simulink model "SimParking"  (R2017b)
settings: Solver=VariableStepAuto  StartTime=0.0  StopTime=1761  RelTol=1e-3
libraries: neural x1111
(part 2 of 60)

== system SimParking/10D- 100 100 100N/Layer 2 ==
  "a{1} " : Inport  PortDimensions=100  SampleTime=1
      mask Display: e = 0.06;c1 = [120 230 180]/255;c2 = ([120 230 180]+0)/(256+128);c3 = ([120 230 180]+128)/(256+128);patch([0 1 1 0],[0 0 1 1],c1);patch([0 1 1 1-e 1-e 0+e],[0 0 1 1-e 0+e 0+e],c2);patch([0 0 1 1-e 0+e 0+e],[0 1 1 1-e 1-e 0+e],c3);plot([0 1 1 0 0],[0 0 1 1 0]);
  Delays 1 : Subsystem
      mask Display: e = 0.06;c1 = [120 150 230]/255;c2 = ([120 150 230]+0)/383;c3 = ([120 150 230]+128)/383;patch([0 1 1 0],[0 0 1 1],c1);patch([0 1 1 1-e 1-e 0+e],[0 0 1 1-e 0+e 0+e],c2);patch([0 0 1 1-e 0+e 0+e],[0 1 1 1-e 1-e 0+e],c3);plot([0 1 1 0 0],[0 0 1 1 0]);disp('0');
  "LW{2,1}" : Subsystem
      mask Display: e = 0.06;c1 = [120 150 230]/255;c2 = ([120 150 230]+0)/383;c3 = ([120 150 230]+128)/383;patch([0 1 1 0],[0 0 1 1],c1);patch([0 1 1 1-e 1-e 0+e],[0 0 1 1-e 0+e 0+e],c2);patch([0 0 1 1-e 0+e 0+e],[0 1 1 1-e 1-e 0+e],c3);plot([0 1 1 0 0],[0 0 1 1 0]);disp('W');
  "b{2}" : Constant  Value=[1.506519516441978456811057185404933989048004150390625;-1.4371919272699462677422843626118265092372894287109375;1.4557843120845770368276816952857188880443572998046875;1.398256717805032689483368812943808734416961669921875;-1.355726258601539502279820226249285042285919189453125;1.359587166719958162275361246429383754730224609375;-1.3155039337803986487784868586459197103977203369140625;-1.3165404698274996153628535466850735247135162353515625;-1.308071637947867404960788917378522455692291259765625;1.27497404400224123577345380908809602260589599609375;1.21468909644321598761962377466261386871337890625;1.1384788543866457555253646205528639256954193115234375;1.0939944737098141747111412769299931824207305908203125;1.1256588211524605203095461547491140663623809814453125;-1.0383506087646006132985121439560316503047943115234375;-1.0161104044606033003361744704307056963443756103515625;-1.0127147984754660825501559884287416934967041015625;0.981450719068787780230422868044115602970123291015625;0.96418217538418382606124623634968884289264678955078125;-0.93556041399205736031063906921190209686756134033203125;-0.87753459394353339195760099755716510117053985595703125;0.87923441768039711785576173497247509658336639404296875;-0.8381966651892593933581565579515881836414337158203125;-0.7681328722554023880064733020844869315624237060546875;-0.75124322279230348886613910508458502590656280517578125;-0.77210854445230181486437004423351027071475982666015625;-0.71873920784606692979679110067081637680530548095703125;-0.70857184198599154623110507600358687341213226318359375;0.6807460268837750572146205740864388644695281982421875;-0.66075686590633697647945155040360987186431884765625;0.62103296432244536884326180370408110320568084716796875;-0.56357924925441860164454510595533065497875213623046875;0.5427900564652194947967700500157661736011505126953125;0.5194764137396343794961239836993627250194549560546875;-0.433960890913997643369981460637063719332218170166015625;0.4821967486735594388136405541445128619670867919921875;0.374432721983393002052054043815587647259235382080078125;-0.37755478669698827598466550625744275748729705810546875;-0.286324330953135197663783628740929998457431793212890625;-0.325139756308971794585005454791826196014881134033203125;0.33221529164236185405201240428141318261623382568359375;-0.1969409792129176162145398620850755833089351654052734375;-0.313389016592093339053093359325430355966091156005859375;-0.192144639089638025186701497659669257700443267822265625;0.2085748723544801064289089254089049063622951507568359375;0.132020705406266258830072501950780861079692840576171875;0.061838232194021347520873632674920372664928436279296875;0.047869259779082858063947725213438388891518115997314453125;-0.006209755679524676941216654313393519259989261627197265625;0.0092266532370322180967026071130021591670811176300048828125;0.004075476244258154252808612483249817159958183765411376953125;-0.06655675450056099118345542819952243007719516754150390625;0.099658129876597112417613288926077075302600860595703125;0.1334403996895525690291606224491260945796966552734375;0.10912476773787938011395226567401550710201263427734375;0.193006691977488042955002356393379159271717071533203125;-0.1454527881073393869026944003053358756005764007568359375;0.185461909127874247094069914965075440704822540283203125;0.2951347935264607702521288956631906330585479736328125;0.3158668243089579608096073570777662098407745361328125;0.294566160388877007481056580218137241899967193603515625;0.380210240619695938324440476208110339939594268798828125;-0.410584596708548243970682278813910670578479766845703125;0.36024445553864425928480841321288608014583587646484375;0.44824097005917129532548415227211080491542816162109375;0.469655642441448251123148338592727668583393096923828125;0.4462810592999779668588189451838843524456024169921875;-0.50698818603659467907363023186917416751384735107421875;0.53901197267530120971201768043101765215396881103515625;-0.54413527250999960127586518865427933633327484130859375 ...(+1616 chars)]
      mask Display: e = 0.06;c1 = [120 150 230]/255;c2 = ([120 150 230]+0)/383;c3 = ([120 150 230]+128)/383;patch([0 1 1 0],[0 0 1 1],c1);patch([0 1 1 1-e 1-e 0+e],[0 0 1 1-e 0+e 0+e],c2);patch([0 0 1 1-e 0+e 0+e],[0 1 1 1-e 1-e 0+e],c3);plot([0 1 1 0 0],[0 0 1 1 0]);disp('b');
  netsum : Sum  Inputs=2  SaturateOnIntegerOverflow=on  InputSameDT=on  OutDataTypeStr=Inherit: Same as first input
      mask Display: e = 0.06;c1 = [120 150 230]/255;c2 = ([120 150 230]+0)/383;c3 = ([120 150 230]+128)/383;patch([0 1 1 0],[0 0 1 1],c1);patch([0 1 1 1-e 1-e 0+e],[0 0 1 1-e 0+e 0+e],c2);patch([0 0 1 1-e 0+e 0+e],[0 1 1 1-e 1-e 0+e],c3);plot([0 1 1 0 0],[0 0 1 1 0]);disp('+');
  tansig : neural/Transfer Functions/tansig
  "a{2}" : Outport  InitialOutput=[0;0;0;0;0;0;0;0;0;0;0;0;0;0;0;0;0;0;0;0;0;0;0;0;0;0;0;0;0;0;0;0;0;0;0;0;0;0;0;0;0;0;0;0;0;0;0;0;0;0;0;0;0;0;0;0;0;0;0;0;0;0;0;0;0;0;0;0;0;0;0;0;0;0;0;0;0;0;0;0;0;0;0;0;0;0;0;0;0;0;0;0;0;0;0;0;0;0;0;0]
      mask Display: e = 0.06;c1 = [120 230 180]/255;c2 = ([120 230 180]+0)/(256+128);c3 = ([120 230 180]+128)/(256+128);patch([0 1 1 0],[0 0 1 1],c1);patch([0 1 1 1-e 1-e 0+e],[0 0 1 1-e 0+e 0+e],c2);patch([0 0 1 1-e 0+e 0+e],[0 1 1 1-e 1-e 0+e],c3);plot([0 1 1 0 0],[0 0 1 1 0]);
  wires:
  "a{1} "/1 -> Delays 1/1("p{2}")
  Delays 1/1("pd{2,1}") -> "LW{2,1}"/1("ad{2,1}")
  "LW{2,1}"/1("lz{2,1}") -> netsum/1
  "b{2}"/1 -> netsum/2
  netsum/1 -> tansig/1
  tansig/1 -> "a{2}"/1

== system SimParking/10D- 100 100 100N/Layer 3 ==
  "a{2} " : Inport  PortDimensions=100  SampleTime=1
      mask Display: e = 0.06;c1 = [120 230 180]/255;c2 = ([120 230 180]+0)/(256+128);c3 = ([120 230 180]+128)/(256+128);patch([0 1 1 0],[0 0 1 1],c1);patch([0 1 1 1-e 1-e 0+e],[0 0 1 1-e 0+e 0+e],c2);patch([0 0 1 1-e 0+e 0+e],[0 1 1 1-e 1-e 0+e],c3);plot([0 1 1 0 0],[0 0 1 1 0]);
  Delays 1 : Subsystem
      mask Display: e = 0.06;c1 = [120 150 230]/255;c2 = ([120 150 230]+0)/383;c3 = ([120 150 230]+128)/383;patch([0 1 1 0],[0 0 1 1],c1);patch([0 1 1 1-e 1-e 0+e],[0 0 1 1-e 0+e 0+e],c2);patch([0 0 1 1-e 0+e 0+e],[0 1 1 1-e 1-e 0+e],c3);plot([0 1 1 0 0],[0 0 1 1 0]);disp('0');
  "LW{3,2}" : Subsystem
      mask Display: e = 0.06;c1 = [120 150 230]/255;c2 = ([120 150 230]+0)/383;c3 = ([120 150 230]+128)/383;patch([0 1 1 0],[0 0 1 1],c1);patch([0 1 1 1-e 1-e 0+e],[0 0 1 1-e 0+e 0+e],c2);patch([0 0 1 1-e 0+e 0+e],[0 1 1 1-e 1-e 0+e],c3);plot([0 1 1 0 0],[0 0 1 1 0]);disp('W');
  "b{3}" : Constant  Value=[-1.4923648462887009191746301439707167446613311767578125;1.4556606612840330416958067871746607124805450439453125;-1.387278892945349451082392988610081374645233154296875;1.4028556882846070497095070095383562147617340087890625;1.345199381926466930536889776703901588916778564453125;1.3532535376566328100267355694086290895938873291015625;-1.30643871860076732360766982310451567173004150390625;-1.2638080303968048934137868855032138526439666748046875;-1.23255646908093563496322531136684119701385498046875;1.230158278997876220017815285245887935161590576171875;1.1333695566611690086489261375390924513339996337890625;-1.1083346531027700176963435296784155070781707763671875;1.11500334128624611906843711039982736110687255859375;1.0878630145011747298866566779906861484050750732421875;1.03732677279241425338796034338884055614471435546875;0.9868555056448837792260064816218800842761993408203125;-1.0240515281041224771030329065979458391666412353515625;-0.9922683117643220640502477181144058704376220703125;-0.94501809355730792550076557745342142879962921142578125;0.870249200573390613300261975382454693317413330078125;-0.8844413015848413550656914594583213329315185546875;-0.8575733682742943120302925308351404964923858642578125;0.84952879702115069449064321815967559814453125;-0.80657709043296066386830034389276988804340362548828125;0.76156012510090598244261173022096045315265655517578125;-0.7558812748899208511232927776291035115718841552734375;0.6629457722732536861798280369839631021022796630859375;-0.67179056724727337357450096533284522593021392822265625;0.64316286659681465298632474514306522905826568603515625;-0.6456362689201016191731241633533500134944915771484375;0.59942726953591651817276897418196313083171844482421875;0.531031473132824505256621705484576523303985595703125;-0.56240602810975437453322456349269486963748931884765625;-0.467483062718826669623695124755613505840301513671875;-0.4667361706627328743479665718041360378265380859375;-0.402814167048342219867862468163366429507732391357421875;0.41212203864621399507228716174722649157047271728515625;0.35396080444632815886762955415179021656513214111328125;0.3871687344655525553349662004620768129825592041015625;-0.31679874280190156721204175482853315770626068115234375;0.2611818277655080233756734742200933396816253662109375;0.238926892331456641738185453505138866603374481201171875;-0.205035418786340295493886287658824585378170013427734375;-0.2129412471957893571161690715598524548113346099853515625;-0.1596725436243604245856175793960574083030223846435546875;-0.139376121918832474033678181513096205890178680419921875;-0.11595637311078853259882492920951335690915584564208984375;0.07992718662413784980191877593824756331741809844970703125;-0.010895986891703089705085716332177980802953243255615234375;0.0183462905284579001763400896152234054170548915863037109375;2.585053176850398811890095751575557869728072546422481536865234375e-05;0.02503199263089939119453219973365776240825653076171875;-0.09852058470632696351998447426012717187404632568359375;-0.10786625805302378633410143038418027572333812713623046875;0.1860671251697297579053014260352938435971736907958984375;0.185573368129740290388696166701265610754489898681640625;-0.241184922099264398287488120331545360386371612548828125;0.20682957005122137861263809099909849464893341064453125;0.263761825941337069156844563622144050896167755126953125;-0.31559160823815213259280199054046534001827239990234375;0.33457105107667317600572687297244556248188018798828125;0.38299603176620011790731723522185347974300384521484375;-0.38103619333580873718148041007225401699542999267578125;0.414633099020468076645329347229562699794769287109375;-0.444740696637884791453387833826127462089061737060546875;-0.449524314866814489466406712381285615265369415283203125;0.474190020993898564416468843774055130779743194580078125;-0.52066741892512291567385318558081053197383880615234375;0.55714918266694135606797999571426771581172943115234375;-0.5895289389142746028227293209056369960308074951171875;-0.61193450214706912593243259834707714617252349853515625 ...(+1575 chars)]
      mask Display: e = 0.06;c1 = [120 150 230]/255;c2 = ([120 150 230]+0)/383;c3 = ([120 150 230]+128)/383;patch([0 1 1 0],[0 0 1 1],c1);patch([0 1 1 1-e 1-e 0+e],[0 0 1 1-e 0+e 0+e],c2);patch([0 0 1 1-e 0+e 0+e],[0 1 1 1-e 1-e 0+e],c3);plot([0 1 1 0 0],[0 0 1 1 0]);disp('b');
  netsum : Sum  Inputs=2  SaturateOnIntegerOverflow=on  InputSameDT=on  OutDataTypeStr=Inherit: Same as first input
      mask Display: e = 0.06;c1 = [120 150 230]/255;c2 = ([120 150 230]+0)/383;c3 = ([120 150 230]+128)/383;patch([0 1 1 0],[0 0 1 1],c1);patch([0 1 1 1-e 1-e 0+e],[0 0 1 1-e 0+e 0+e],c2);patch([0 0 1 1-e 0+e 0+e],[0 1 1 1-e 1-e 0+e],c3);plot([0 1 1 0 0],[0 0 1 1 0]);disp('+');
  tansig : neural/Transfer Functions/tansig
  "a{3}" : Outport  InitialOutput=[0;0;0;0;0;0;0;0;0;0;0;0;0;0;0;0;0;0;0;0;0;0;0;0;0;0;0;0;0;0;0;0;0;0;0;0;0;0;0;0;0;0;0;0;0;0;0;0;0;0;0;0;0;0;0;0;0;0;0;0;0;0;0;0;0;0;0;0;0;0;0;0;0;0;0;0;0;0;0;0;0;0;0;0;0;0;0;0;0;0;0;0;0;0;0;0;0;0;0;0]
      mask Display: e = 0.06;c1 = [120 230 180]/255;c2 = ([120 230 180]+0)/(256+128);c3 = ([120 230 180]+128)/(256+128);patch([0 1 1 0],[0 0 1 1],c1);patch([0 1 1 1-e 1-e 0+e],[0 0 1 1-e 0+e 0+e],c2);patch([0 0 1 1-e 0+e 0+e],[0 1 1 1-e 1-e 0+e],c3);plot([0 1 1 0 0],[0 0 1 1 0]);
  wires:
  "a{2} "/1 -> Delays 1/1("p{3}")
  Delays 1/1("pd{3,2}") -> "LW{3,2}"/1("ad{3,2}")
  "LW{3,2}"/1("lz{3,2}") -> netsum/1
  "b{3}"/1 -> netsum/2
  netsum/1 -> tansig/1
  tansig/1 -> "a{3}"/1

== system SimParking/10D- 100 100 100N/Layer 4 ==
  "a{3} " : Inport  PortDimensions=100  SampleTime=1
      mask Display: e = 0.06;c1 = [120 230 180]/255;c2 = ([120 230 180]+0)/(256+128);c3 = ([120 230 180]+128)/(256+128);patch([0 1 1 0],[0 0 1 1],c1);patch([0 1 1 1-e 1-e 0+e],[0 0 1 1-e 0+e 0+e],c2);patch([0 0 1 1-e 0+e 0+e],[0 1 1 1-e 1-e 0+e],c3);plot([0 1 1 0 0],[0 0 1 1 0]);
  Delays 1 : Subsystem
      mask Display: e = 0.06;c1 = [120 150 230]/255;c2 = ([120 150 230]+0)/383;c3 = ([120 150 230]+128)/383;patch([0 1 1 0],[0 0 1 1],c1);patch([0 1 1 1-e 1-e 0+e],[0 0 1 1-e 0+e 0+e],c2);patch([0 0 1 1-e 0+e 0+e],[0 1 1 1-e 1-e 0+e],c3);plot([0 1 1 0 0],[0 0 1 1 0]);disp('0');
  "LW{4,3}" : Subsystem
      mask Display: e = 0.06;c1 = [120 150 230]/255;c2 = ([120 150 230]+0)/383;c3 = ([120 150 230]+128)/383;patch([0 1 1 0],[0 0 1 1],c1);patch([0 1 1 1-e 1-e 0+e],[0 0 1 1-e 0+e 0+e],c2);patch([0 0 1 1-e 0+e 0+e],[0 1 1 1-e 1-e 0+e],c3);plot([0 1 1 0 0],[0 0 1 1 0]);disp('W');
  "b{4}" : Constant  Value=[0.90458221227192170399433734928607009351253509521484375;-0.09842194346834050311390029719404992647469043731689453125;-0.8300561660103167316293593103182502090930938720703125]
      mask Display: e = 0.06;c1 = [120 150 230]/255;c2 = ([120 150 230]+0)/383;c3 = ([120 150 230]+128)/383;patch([0 1 1 0],[0 0 1 1],c1);patch([0 1 1 1-e 1-e 0+e],[0 0 1 1-e 0+e 0+e],c2);patch([0 0 1 1-e 0+e 0+e],[0 1 1 1-e 1-e 0+e],c3);plot([0 1 1 0 0],[0 0 1 1 0]);disp('b');
  netsum : Sum  Inputs=2  SaturateOnIntegerOverflow=on  InputSameDT=on  OutDataTypeStr=Inherit: Same as first input
      mask Display: e = 0.06;c1 = [120 150 230]/255;c2 = ([120 150 230]+0)/383;c3 = ([120 150 230]+128)/383;patch([0 1 1 0],[0 0 1 1],c1);patch([0 1 1 1-e 1-e 0+e],[0 0 1 1-e 0+e 0+e],c2);patch([0 0 1 1-e 0+e 0+e],[0 1 1 1-e 1-e 0+e],c3);plot([0 1 1 0 0],[0 0 1 1 0]);disp('+');
  purelin : neural/Transfer Functions/purelin
  "a{4}" : Outport  InitialOutput=[0;0;0]
      mask Display: e = 0.06;c1 = [120 230 180]/255;c2 = ([120 230 180]+0)/(256+128);c3 = ([120 230 180]+128)/(256+128);patch([0 1 1 0],[0 0 1 1],c1);patch([0 1 1 1-e 1-e 0+e],[0 0 1 1-e 0+e 0+e],c2);patch([0 0 1 1-e 0+e 0+e],[0 1 1 1-e 1-e 0+e],c3);plot([0 1 1 0 0],[0 0 1 1 0]);
  wires:
  "a{3} "/1 -> Delays 1/1("p{4}")
  Delays 1/1("pd{4,3}") -> "LW{4,3}"/1("ad{4,3}")
  "LW{4,3}"/1("lz{4,3}") -> netsum/1
  "b{4}"/1 -> netsum/2
  netsum/1 -> purelin/1
  purelin/1 -> "a{4}"/1

== system SimParking/10D- 100 100 100N/Process Input 1 ==
  x : Inport  PortDimensions=9  SampleTime=1
      mask Display: e = 0.06;c1 = [120 230 180]/255;c2 = ([120 230 180]+0)/(256+128);c3 = ([120 230 180]+128)/(256+128);patch([0 1 1 0],[0 0 1 1],c1);patch([0 1 1 1-e 1-e 0+e],[0 0 1 1-e 0+e 0+e],c2);patch([0 0 1 1-e 0+e 0+e],[0 1 1 1-e 1-e 0+e],c3);plot([0 1 1 0 0],[0 0 1 1 0]);
  mapminmax : neural/Processing Functions/mapminmax  xmin=[0;-0.00100000000000000002081668171172;-0.969999999999999973354647408996;-0.0367373000000000005105249556436;0;0;0;0;0]  xmax=[1;4.75300000000000011368683772162;0;1.12596000000000007190692485892;4.47799999999999975841546984157;1;1;1;1]  ymin=-1  ymax=1
  p : Outport  PortDimensions=9  SampleTime=1
      mask Display: e = 0.06;c1 = [120 230 180]/255;c2 = ([120 230 180]+0)/(256+128);c3 = ([120 230 180]+128)/(256+128);patch([0 1 1 0],[0 0 1 1],c1);patch([0 1 1 1-e 1-e 0+e],[0 0 1 1-e 0+e 0+e],c2);patch([0 0 1 1-e 0+e 0+e],[0 1 1 1-e 1-e 0+e],c3);plot([0 1 1 0 0],[0 0 1 1 0]);
  wires:
  x/1 -> mapminmax/1
  mapminmax/1 -> p/1

== system SimParking/10D- 100 100 100N/Process Output 1 ==
  a : Inport  PortDimensions=3  SampleTime=1
      mask Display: e = 0.06;c1 = [120 230 180]/255;c2 = ([120 230 180]+0)/(256+128);c3 = ([120 230 180]+128)/(256+128);patch([0 1 1 0],[0 0 1 1],c1);patch([0 1 1 1-e 1-e 0+e],[0 0 1 1-e 0+e 0+e],c2);patch([0 0 1 1-e 0+e 0+e],[0 1 1 1-e 1-e 0+e],c3);plot([0 1 1 0 0],[0 0 1 1 0]);
  mapminmax_reverse : neural/Processing Functions/mapminmax_reverse  xmin=[-0.142810999999999993503863038313;-0.169776000000000010237144465464;0]  xmax=[0.231192000000000008608225243734;0.179999999999999993338661852249;1]  ymin=-1  ymax=1
  y : Outport  PortDimensions=3  SampleTime=1
      mask Display: e = 0.06;c1 = [120 230 180]/255;c2 = ([120 230 180]+0)/(256+128);c3 = ([120 230 180]+128)/(256+128);patch([0 1 1 0],[0 0 1 1],c1);patch([0 1 1 1-e 1-e 0+e],[0 0 1 1-e 0+e 0+e],c2);patch([0 0 1 1-e 0+e 0+e],[0 1 1 1-e 1-e 0+e],c3);plot([0 1 1 0 0],[0 0 1 1 0]);
  wires:
  a/1 -> mapminmax_reverse/1
  mapminmax_reverse/1 -> y/1

== system SimParking/10D- 50 50 50 N/Layer 1 ==
  "p{1}" : Inport  PortDimensions=9  SampleTime=1
      mask Display: e = 0.06;c1 = [120 230 180]/255;c2 = ([120 230 180]+0)/(256+128);c3 = ([120 230 180]+128)/(256+128);patch([0 1 1 0],[0 0 1 1],c1);patch([0 1 1 1-e 1-e 0+e],[0 0 1 1-e 0+e 0+e],c2);patch([0 0 1 1-e 0+e 0+e],[0 1 1 1-e 1-e 0+e],c3);plot([0 1 1 0 0],[0 0 1 1 0]);
  Delays 1 : Subsystem
      mask Display: e = 0.06;c1 = [120 150 230]/255;c2 = ([120 150 230]+0)/383;c3 = ([120 150 230]+128)/383;patch([0 1 1 0],[0 0 1 1],c1);patch([0 1 1 1-e 1-e 0+e],[0 0 1 1-e 0+e 0+e],c2);patch([0 0 1 1-e 0+e 0+e],[0 1 1 1-e 1-e 0+e],c3);plot([0 1 1 0 0],[0 0 1 1 0]);disp('1-10');
  "IW{1,1}" : Subsystem
      mask Display: e = 0.06;c1 = [120 150 230]/255;c2 = ([120 150 230]+0)/383;c3 = ([120 150 230]+128)/383;patch([0 1 1 0],[0 0 1 1],c1);patch([0 1 1 1-e 1-e 0+e],[0 0 1 1-e 0+e 0+e],c2);patch([0 0 1 1-e 0+e 0+e],[0 1 1 1-e 1-e 0+e],c3);plot([0 1 1 0 0],[0 0 1 1 0]);disp('W');
  "b{1}" : Constant  Value=[1.4993079978726011614043045483413152396678924560546875;1.3542460844650008322531675730715505778789520263671875;1.3907982191069423461016185683547519147396087646484375;1.308490195985559711999712817487306892871856689453125;1.1405229519144501892924381536431610584259033203125;1.2489696034493473764115378799033351242542266845703125;-1.015338567140214198758485508733429014682769775390625;1.084892394960385697544325012131594121456146240234375;-1.020033929194558819375515668070875108242034912109375;-0.9167754303620501143967658208566717803478240966796875;0.856095643214190626935078398673795163631439208984375;0.9575612333326513070375085590058006346225738525390625;-0.74290663708967452638631812078529037535190582275390625;0.7899760190835694029232172397314570844173431396484375;-0.6791269114960456487750661835889331996440887451171875;0.494812201714843580280245305402786470949649810791015625;-0.48259957168908951263830431344103999435901641845703125;0.466592017646469958691568535869009792804718017578125;0.44091398797479330884385717581608332693576812744140625;-0.3463473555985283613978253924869932234287261962890625;0.320059588629600322295942760320031084120273590087890625;-0.1916844930808605240724062923618475906550884246826171875;-0.236667310543505593489754801339586265385150909423828125;-0.05896019531653860779041309569947770796716213226318359375;-0.0054578617790423666900068155882763676345348358154296875;-0.09436511622671876764467668863289873115718364715576171875;0.056430351654014533624437177650179364718496799468994140625;-0.09151564734804855383298871629449422471225261688232421875;-0.198838769579198493264726721463375724852085113525390625;-0.2243404452870361442951008257296052761375904083251953125;-0.283546912314165677759802974833291955292224884033203125;-0.32550350432140728873520174602163024246692657470703125;-0.5355126930982463395736203892738558351993560791015625;0.58564933843603272922706537428894080221652984619140625;-0.59827548757695281356205896372557617723941802978515625;-0.64002381064156310674917449432541616261005401611328125;0.7358374465386725571391934863640926778316497802734375;-0.727636428195794326967416054685600101947784423828125;-0.78562713595295130541984462979598902165889739990234375;0.90797256959115346663935497417696751654148101806640625;0.8552038045728507231757475892663933336734771728515625;1.05149309203325902473125097458250820636749267578125;0.99187140224879410954628156105172820389270782470703125;-1.1346964494664690814573759780614636838436126708984375;-1.21690924045593273916665566503070294857025146484375;1.2315265799796242252028832808719016611576080322265625;-1.295898025840918510454002898768521845340728759765625;1.4632848771443620616850012083887122571468353271484375;1.4344329471441412682253258026321418583393096923828125;-1.4858519669939604934683075043722055852413177490234375]
      mask Display: e = 0.06;c1 = [120 150 230]/255;c2 = ([120 150 230]+0)/383;c3 = ([120 150 230]+128)/383;patch([0 1 1 0],[0 0 1 1],c1);patch([0 1 1 1-e 1-e 0+e],[0 0 1 1-e 0+e 0+e],c2);patch([0 0 1 1-e 0+e 0+e],[0 1 1 1-e 1-e 0+e],c3);plot([0 1 1 0 0],[0 0 1 1 0]);disp('b');
  netsum : Sum  Inputs=2  SaturateOnIntegerOverflow=on  InputSameDT=on  OutDataTypeStr=Inherit: Same as first input
      mask Display: e = 0.06;c1 = [120 150 230]/255;c2 = ([120 150 230]+0)/383;c3 = ([120 150 230]+128)/383;patch([0 1 1 0],[0 0 1 1],c1);patch([0 1 1 1-e 1-e 0+e],[0 0 1 1-e 0+e 0+e],c2);patch([0 0 1 1-e 0+e 0+e],[0 1 1 1-e 1-e 0+e],c3);plot([0 1 1 0 0],[0 0 1 1 0]);disp('+');
  tansig : neural/Transfer Functions/tansig
  "a{1}" : Outport  InitialOutput=[0;0;0;0;0;0;0;0;0;0;0;0;0;0;0;0;0;0;0;0;0;0;0;0;0;0;0;0;0;0;0;0;0;0;0;0;0;0;0;0;0;0;0;0;0;0;0;0;0;0]
      mask Display: e = 0.06;c1 = [120 230 180]/255;c2 = ([120 230 180]+0)/(256+128);c3 = ([120 230 180]+128)/(256+128);patch([0 1 1 0],[0 0 1 1],c1);patch([0 1 1 1-e 1-e 0+e],[0 0 1 1-e 0+e 0+e],c2);patch([0 0 1 1-e 0+e 0+e],[0 1 1 1-e 1-e 0+e],c3);plot([0 1 1 0 0],[0 0 1 1 0]);
  wires:
  "p{1}"/1 -> Delays 1/1("p{1}")
  Delays 1/1("pd{1,1}") -> "IW{1,1}"/1("pd{1,1}")
  "IW{1,1}"/1("iz{1,1}") -> netsum/1
  "b{1}"/1 -> netsum/2
  netsum/1 -> tansig/1
  tansig/1 -> "a{1}"/1

== system SimParking/10D- 50 50 50 N/Layer 2 ==
  "a{1} " : Inport  PortDimensions=50  SampleTime=1
      mask Display: e = 0.06;c1 = [120 230 180]/255;c2 = ([120 230 180]+0)/(256+128);c3 = ([120 230 180]+128)/(256+128);patch([0 1 1 0],[0 0 1 1],c1);patch([0 1 1 1-e 1-e 0+e],[0 0 1 1-e 0+e 0+e],c2);patch([0 0 1 1-e 0+e 0+e],[0 1 1 1-e 1-e 0+e],c3);plot([0 1 1 0 0],[0 0 1 1 0]);
  Delays 1 : Subsystem
      mask Display: e = 0.06;c1 = [120 150 230]/255;c2 = ([120 150 230]+0)/383;c3 = ([120 150 230]+128)/383;patch([0 1 1 0],[0 0 1 1],c1);patch([0 1 1 1-e 1-e 0+e],[0 0 1 1-e 0+e 0+e],c2);patch([0 0 1 1-e 0+e 0+e],[0 1 1 1-e 1-e 0+e],c3);plot([0 1 1 0 0],[0 0 1 1 0]);disp('0');
  "LW{2,1}" : Subsystem
      mask Display: e = 0.06;c1 = [120 150 230]/255;c2 = ([120 150 230]+0)/383;c3 = ([120 150 230]+128)/383;patch([0 1 1 0],[0 0 1 1],c1);patch([0 1 1 1-e 1-e 0+e],[0 0 1 1-e 0+e 0+e],c2);patch([0 0 1 1-e 0+e 0+e],[0 1 1 1-e 1-e 0+e],c3);plot([0 1 1 0 0],[0 0 1 1 0]);disp('W');
  "b{2}" : Constant  Value=[-1.5558665204435995210729970494867302477359771728515625;1.4982971009886369984087650664150714874267578125;-1.398393996236940939326132138376124203205108642578125;-1.3273992334518889268935026848339475691318511962890625;1.331855793684081579186795352143235504627227783203125;-1.19211217156784865522922700620256364345550537109375;1.0559487576740662628793643307290039956569671630859375;-1.121692647798080866294867519172839820384979248046875;1.0445365176782070992800299791269935667514801025390625;0.90548194447669538842404790557338856160640716552734375;-0.9424410267084353254318784820497967302799224853515625;0.8701887279449198597802705990034155547618865966796875;-0.7881628233449340381611136763240210711956024169921875;0.79938561743112435120650616227067075669765472412109375;-0.6666562963735012115051858927472494542598724365234375;0.60696755195962115436714157112874090671539306640625;-0.51477148341905898387693696349742822349071502685546875;-0.43892883434105878226461072699748910963535308837890625;-0.353327933690762652219063966185785830020904541015625;-0.32253740194440883026771871300297789275646209716796875;-0.289050561394564475836688188792322762310504913330078125;0.14840099014217378314839379527256824076175689697265625;-0.1103284356851219893957960493935388512909412384033203125;0.143926574806760243507852692346205003559589385986328125;0.0599788026191515888374539144933805800974369049072265625;0.08142853545393748115888143956908606924116611480712890625;0.1229638467831936921026425579839269630610942840576171875;-0.213254189066676980157666321247234009206295013427734375;0.18447471393838676956278277430101297795772552490234375;-0.33352367076396571832219706266187131404876708984375;0.371070208556163960711415938931168057024478912353515625;0.423289852743953198821458272504969500005245208740234375;-0.4492709015673082006969707435928285121917724609375;-0.547250176899218399029223292018286883831024169921875;-0.58020729285361183347191627035499550402164459228515625;-0.6070177510070691173638124382705427706241607666015625;0.7256602590846374933875040369457565248012542724609375;-0.7790281573144710591805051080882549285888671875;0.84831525272277563676226463940110988914966583251953125;-0.93043991258574665348390908548026345670223236083984375;-0.98385232091231411555298791427048854529857635498046875;1.09921105202476088180674196337349712848663330078125;1.1161630097631860536466774647124111652374267578125;-1.1849406049304025412283181140082888305187225341796875;-1.2393061180855513558896063841530121862888336181640625;1.289831570647042013888494693674147129058837890625;1.39798535801373358111732159159146249294281005859375;1.4649827348859807418790524025098420679569244384765625;-1.4537989856769424346083496857318095862865447998046875;1.457395770530155232336255721747875213623046875]
      mask Display: e = 0.06;c1 = [120 150 230]/255;c2 = ([120 150 230]+0)/383;c3 = ([120 150 230]+128)/383;patch([0 1 1 0],[0 0 1 1],c1);patch([0 1 1 1-e 1-e 0+e],[0 0 1 1-e 0+e 0+e],c2);patch([0 0 1 1-e 0+e 0+e],[0 1 1 1-e 1-e 0+e],c3);plot([0 1 1 0 0],[0 0 1 1 0]);disp('b');
  netsum : Sum  Inputs=2  SaturateOnIntegerOverflow=on  InputSameDT=on  OutDataTypeStr=Inherit: Same as first input
      mask Display: e = 0.06;c1 = [120 150 230]/255;c2 = ([120 150 230]+0)/383;c3 = ([120 150 230]+128)/383;patch([0 1 1 0],[0 0 1 1],c1);patch([0 1 1 1-e 1-e 0+e],[0 0 1 1-e 0+e 0+e],c2);patch([0 0 1 1-e 0+e 0+e],[0 1 1 1-e 1-e 0+e],c3);plot([0 1 1 0 0],[0 0 1 1 0]);disp('+');
  tansig : neural/Transfer Functions/tansig
  "a{2}" : Outport  InitialOutput=[0;0;0;0;0;0;0;0;0;0;0;0;0;0;0;0;0;0;0;0;0;0;0;0;0;0;0;0;0;0;0;0;0;0;0;0;0;0;0;0;0;0;0;0;0;0;0;0;0;0]
      mask Display: e = 0.06;c1 = [120 230 180]/255;c2 = ([120 230 180]+0)/(256+128);c3 = ([120 230 180]+128)/(256+128);patch([0 1 1 0],[0 0 1 1],c1);patch([0 1 1 1-e 1-e 0+e],[0 0 1 1-e 0+e 0+e],c2);patch([0 0 1 1-e 0+e 0+e],[0 1 1 1-e 1-e 0+e],c3);plot([0 1 1 0 0],[0 0 1 1 0]);
  wires:
  "a{1} "/1 -> Delays 1/1("p{2}")
  Delays 1/1("pd{2,1}") -> "LW{2,1}"/1("ad{2,1}")
  "LW{2,1}"/1("lz{2,1}") -> netsum/1
  "b{2}"/1 -> netsum/2
  netsum/1 -> tansig/1
  tansig/1 -> "a{2}"/1

== system SimParking/10D- 50 50 50 N/Layer 3 ==
  "a{2} " : Inport  PortDimensions=50  SampleTime=1
      mask Display: e = 0.06;c1 = [120 230 180]/255;c2 = ([120 230 180]+0)/(256+128);c3 = ([120 230 180]+128)/(256+128);patch([0 1 1 0],[0 0 1 1],c1);patch([0 1 1 1-e 1-e 0+e],[0 0 1 1-e 0+e 0+e],c2);patch([0 0 1 1-e 0+e 0+e],[0 1 1 1-e 1-e 0+e],c3);plot([0 1 1 0 0],[0 0 1 1 0]);
  Delays 1 : Subsystem
      mask Display: e = 0.06;c1 = [120 150 230]/255;c2 = ([120 150 230]+0)/383;c3 = ([120 150 230]+128)/383;patch([0 1 1 0],[0 0 1 1],c1);patch([0 1 1 1-e 1-e 0+e],[0 0 1 1-e 0+e 0+e],c2);patch([0 0 1 1-e 0+e 0+e],[0 1 1 1-e 1-e 0+e],c3);plot([0 1 1 0 0],[0 0 1 1 0]);disp('0');
  "LW{3,2}" : Subsystem
      mask Display: e = 0.06;c1 = [120 150 230]/255;c2 = ([120 150 230]+0)/383;c3 = ([120 150 230]+128)/383;patch([0 1 1 0],[0 0 1 1],c1);patch([0 1 1 1-e 1-e 0+e],[0 0 1 1-e 0+e 0+e],c2);patch([0 0 1 1-e 0+e 0+e],[0 1 1 1-e 1-e 0+e],c3);plot([0 1 1 0 0],[0 0 1 1 0]);disp('W');
  "b{3}" : Constant  Value=[1.515937439088637095352396499947644770145416259765625;-1.4591060352060052363043496370664797723293304443359375;1.402501298546458219362875752267427742481231689453125;1.35231474348406965901858711731620132923126220703125;1.3210483483525958803284083842299878597259521484375;1.1951895307913205090954988918383605778217315673828125;1.137618485958335146079889454995281994342803955078125;1.0967895366618092278798712868592701852321624755859375;1.0231405797009192060187388051417656242847442626953125;0.96470855530445176473364199409843422472476959228515625;-0.8925616182950903976234258152544498443603515625;0.8056045386011982945007048328989185392856597900390625;-0.79787830142570104197119462696718983352184295654296875;-0.760535392456034298191980269621126353740692138671875;0.62558343059505061578562390423030592501163482666015625;-0.59360828487597672165065887384116649627685546875;0.456763196622117728651346624246798455715179443359375;-0.46567858339936230027689134658430702984333038330078125;-0.39904208695783782712140919102239422500133514404296875;-0.372573670495543740610600025320309214293956756591796875;0.2789671805495050893597408503410406410694122314453125;-0.18863115738773839069608584395609796047210693359375;-0.182947515142232786100606745094410143792629241943359375;-0.08870676414596283254621056357791530899703502655029296875;-0.01038617128180646144441912070988109917379915714263916015625;0.025089060189266453038126059027490555308759212493896484375;0.1258372426746467154234920826638699509203433990478515625;-0.1990483219836979567052281936412327922880649566650390625;-0.2152768186913570913620930014076293446123600006103515625;0.260489277743027269895748077033204026520252227783203125;-0.340461166993566044514096802231506444513797760009765625;-0.327031805839900935328756759190582670271396636962890625;0.45878797737122034572365691929007880389690399169921875;0.54139635945644248860020297797746025025844573974609375;-0.6247835473444809384346854130853898823261260986328125;-0.6429884088792732210748681609402410686016082763671875;-0.7429951106886398815021266273106448352336883544921875;-0.82386680640117904150798722184845246374607086181640625;0.84786986584271362143994110738276503980159759521484375;0.90637180038879616716940290643833577632904052734375;-1.013641540014472042230408987961709499359130859375;0.9973101180982240077099731934140436351299285888671875;1.12217992658560117291699498309753835201263427734375;-1.10207380001778876277285235119052231311798095703125;1.2026391021060029995481954756542108952999114990234375;-1.233423413906584276134026367799378931522369384765625;1.2624782564224250602791244091349653899669647216796875;1.420883396647349083963263183250091969966888427734375;1.4837410308911866962944259284995496273040771484375;1.5200204987602836670390615836367942392826080322265625]
      mask Display: e = 0.06;c1 = [120 150 230]/255;c2 = ([120 150 230]+0)/383;c3 = ([120 150 230]+128)/383;patch([0 1 1 0],[0 0 1 1],c1);patch([0 1 1 1-e 1-e 0+e],[0 0 1 1-e 0+e 0+e],c2);patch([0 0 1 1-e 0+e 0+e],[0 1 1 1-e 1-e 0+e],c3);plot([0 1 1 0 0],[0 0 1 1 0]);disp('b');
  netsum : Sum  Inputs=2  SaturateOnIntegerOverflow=on  InputSameDT=on  OutDataTypeStr=Inherit: Same as first input
      mask Display: e = 0.06;c1 = [120 150 230]/255;c2 = ([120 150 230]+0)/383;c3 = ([120 150 230]+128)/383;patch([0 1 1 0],[0 0 1 1],c1);patch([0 1 1 1-e 1-e 0+e],[0 0 1 1-e 0+e 0+e],c2);patch([0 0 1 1-e 0+e 0+e],[0 1 1 1-e 1-e 0+e],c3);plot([0 1 1 0 0],[0 0 1 1 0]);disp('+');
  tansig : neural/Transfer Functions/tansig
  "a{3}" : Outport  InitialOutput=[0;0;0;0;0;0;0;0;0;0;0;0;0;0;0;0;0;0;0;0;0;0;0;0;0;0;0;0;0;0;0;0;0;0;0;0;0;0;0;0;0;0;0;0;0;0;0;0;0;0]
      mask Display: e = 0.06;c1 = [120 230 180]/255;c2 = ([120 230 180]+0)/(256+128);c3 = ([120 230 180]+128)/(256+128);patch([0 1 1 0],[0 0 1 1],c1);patch([0 1 1 1-e 1-e 0+e],[0 0 1 1-e 0+e 0+e],c2);patch([0 0 1 1-e 0+e 0+e],[0 1 1 1-e 1-e 0+e],c3);plot([0 1 1 0 0],[0 0 1 1 0]);
  wires:
  "a{2} "/1 -> Delays 1/1("p{3}")
  Delays 1/1("pd{3,2}") -> "LW{3,2}"/1("ad{3,2}")
  "LW{3,2}"/1("lz{3,2}") -> netsum/1
  "b{3}"/1 -> netsum/2
  netsum/1 -> tansig/1
  tansig/1 -> "a{3}"/1

== system SimParking/10D- 50 50 50 N/Layer 4 ==
  "a{3} " : Inport  PortDimensions=50  SampleTime=1
      mask Display: e = 0.06;c1 = [120 230 180]/255;c2 = ([120 230 180]+0)/(256+128);c3 = ([120 230 180]+128)/(256+128);patch([0 1 1 0],[0 0 1 1],c1);patch([0 1 1 1-e 1-e 0+e],[0 0 1 1-e 0+e 0+e],c2);patch([0 0 1 1-e 0+e 0+e],[0 1 1 1-e 1-e 0+e],c3);plot([0 1 1 0 0],[0 0 1 1 0]);
  Delays 1 : Subsystem
      mask Display: e = 0.06;c1 = [120 150 230]/255;c2 = ([120 150 230]+0)/383;c3 = ([120 150 230]+128)/383;patch([0 1 1 0],[0 0 1 1],c1);patch([0 1 1 1-e 1-e 0+e],[0 0 1 1-e 0+e 0+e],c2);patch([0 0 1 1-e 0+e 0+e],[0 1 1 1-e 1-e 0+e],c3);plot([0 1 1 0 0],[0 0 1 1 0]);disp('0');
  "LW{4,3}" : Subsystem
      mask Display: e = 0.06;c1 = [120 150 230]/255;c2 = ([120 150 230]+0)/383;c3 = ([120 150 230]+128)/383;patch([0 1 1 0],[0 0 1 1],c1);patch([0 1 1 1-e 1-e 0+e],[0 0 1 1-e 0+e 0+e],c2);patch([0 0 1 1-e 0+e 0+e],[0 1 1 1-e 1-e 0+e],c3);plot([0 1 1 0 0],[0 0 1 1 0]);disp('W');
  "b{4}" : Constant  Value=[0.6652378092665769404590037083835341036319732666015625;-0.803099085688466107768590518389828503131866455078125;0.99076145875711330024415701700490899384021759033203125]
      mask Display: e = 0.06;c1 = [120 150 230]/255;c2 = ([120 150 230]+0)/383;c3 = ([120 150 230]+128)/383;patch([0 1 1 0],[0 0 1 1],c1);patch([0 1 1 1-e 1-e 0+e],[0 0 1 1-e 0+e 0+e],c2);patch([0 0 1 1-e 0+e 0+e],[0 1 1 1-e 1-e 0+e],c3);plot([0 1 1 0 0],[0 0 1 1 0]);disp('b');
  netsum : Sum  Inputs=2  SaturateOnIntegerOverflow=on  InputSameDT=on  OutDataTypeStr=Inherit: Same as first input
      mask Display: e = 0.06;c1 = [120 150 230]/255;c2 = ([120 150 230]+0)/383;c3 = ([120 150 230]+128)/383;patch([0 1 1 0],[0 0 1 1],c1);patch([0 1 1 1-e 1-e 0+e],[0 0 1 1-e 0+e 0+e],c2);patch([0 0 1 1-e 0+e 0+e],[0 1 1 1-e 1-e 0+e],c3);plot([0 1 1 0 0],[0 0 1 1 0]);disp('+');
  purelin : neural/Transfer Functions/purelin
  "a{4}" : Outport  InitialOutput=[0;0;0]
      mask Display: e = 0.06;c1 = [120 230 180]/255;c2 = ([120 230 180]+0)/(256+128);c3 = ([120 230 180]+128)/(256+128);patch([0 1 1 0],[0 0 1 1],c1);patch([0 1 1 1-e 1-e 0+e],[0 0 1 1-e 0+e 0+e],c2);patch([0 0 1 1-e 0+e 0+e],[0 1 1 1-e 1-e 0+e],c3);plot([0 1 1 0 0],[0 0 1 1 0]);
  wires:
  "a{3} "/1 -> Delays 1/1("p{4}")
  Delays 1/1("pd{4,3}") -> "LW{4,3}"/1("ad{4,3}")
  "LW{4,3}"/1("lz{4,3}") -> netsum/1
  "b{4}"/1 -> netsum/2
  netsum/1 -> purelin/1
  purelin/1 -> "a{4}"/1

== system SimParking/10D- 50 50 50 N/Process Input 1 ==
  x : Inport  PortDimensions=9  SampleTime=1
      mask Display: e = 0.06;c1 = [120 230 180]/255;c2 = ([120 230 180]+0)/(256+128);c3 = ([120 230 180]+128)/(256+128);patch([0 1 1 0],[0 0 1 1],c1);patch([0 1 1 1-e 1-e 0+e],[0 0 1 1-e 0+e 0+e],c2);patch([0 0 1 1-e 0+e 0+e],[0 1 1 1-e 1-e 0+e],c3);plot([0 1 1 0 0],[0 0 1 1 0]);
  mapminmax : neural/Processing Functions/mapminmax  xmin=[0;-0.00100000000000000002081668171172;-0.969999999999999973354647408996;-0.0367373000000000005105249556436;0;0;0;0;0]  xmax=[1;4.75300000000000011368683772162;0;1.12596000000000007190692485892;4.47799999999999975841546984157;1;1;1;1]  ymin=-1  ymax=1
  p : Outport  PortDimensions=9  SampleTime=1
      mask Display: e = 0.06;c1 = [120 230 180]/255;c2 = ([120 230 180]+0)/(256+128);c3 = ([120 230 180]+128)/(256+128);patch([0 1 1 0],[0 0 1 1],c1);patch([0 1 1 1-e 1-e 0+e],[0 0 1 1-e 0+e 0+e],c2);patch([0 0 1 1-e 0+e 0+e],[0 1 1 1-e 1-e 0+e],c3);plot([0 1 1 0 0],[0 0 1 1 0]);
  wires:
  x/1 -> mapminmax/1
  mapminmax/1 -> p/1

== system SimParking/10D- 50 50 50 N/Process Output 1 ==
  a : Inport  PortDimensions=3  SampleTime=1
      mask Display: e = 0.06;c1 = [120 230 180]/255;c2 = ([120 230 180]+0)/(256+128);c3 = ([120 230 180]+128)/(256+128);patch([0 1 1 0],[0 0 1 1],c1);patch([0 1 1 1-e 1-e 0+e],[0 0 1 1-e 0+e 0+e],c2);patch([0 0 1 1-e 0+e 0+e],[0 1 1 1-e 1-e 0+e],c3);plot([0 1 1 0 0],[0 0 1 1 0]);
  mapminmax_reverse : neural/Processing Functions/mapminmax_reverse  xmin=[-0.142810999999999993503863038313;-0.169776000000000010237144465464;0]  xmax=[0.231192000000000008608225243734;0.179999999999999993338661852249;1]  ymin=-1  ymax=1
  y : Outport  PortDimensions=3  SampleTime=1
      mask Display: e = 0.06;c1 = [120 230 180]/255;c2 = ([120 230 180]+0)/(256+128);c3 = ([120 230 180]+128)/(256+128);patch([0 1 1 0],[0 0 1 1],c1);patch([0 1 1 1-e 1-e 0+e],[0 0 1 1-e 0+e 0+e],c2);patch([0 0 1 1-e 0+e 0+e],[0 1 1 1-e 1-e 0+e],c3);plot([0 1 1 0 0],[0 0 1 1 0]);
  wires:
  a/1 -> mapminmax_reverse/1
  mapminmax_reverse/1 -> y/1

== system SimParking/BestNet- 10 delays -100 100 hidden neurons/Layer 1 ==
  "p{1}" : Inport  PortDimensions=9  SampleTime=1
      mask Display: e = 0.06;c1 = [120 230 180]/255;c2 = ([120 230 180]+0)/(256+128);c3 = ([120 230 180]+128)/(256+128);patch([0 1 1 0],[0 0 1 1],c1);patch([0 1 1 1-e 1-e 0+e],[0 0 1 1-e 0+e 0+e],c2);patch([0 0 1 1-e 0+e 0+e],[0 1 1 1-e 1-e 0+e],c3);plot([0 1 1 0 0],[0 0 1 1 0]);
  Delays 1 : Subsystem
      mask Display: e = 0.06;c1 = [120 150 230]/255;c2 = ([120 150 230]+0)/383;c3 = ([120 150 230]+128)/383;patch([0 1 1 0],[0 0 1 1],c1);patch([0 1 1 1-e 1-e 0+e],[0 0 1 1-e 0+e 0+e],c2);patch([0 0 1 1-e 0+e 0+e],[0 1 1 1-e 1-e 0+e],c3);plot([0 1 1 0 0],[0 0 1 1 0]);disp('1-10');
  "IW{1,1}" : Subsystem
      mask Display: e = 0.06;c1 = [120 150 230]/255;c2 = ([120 150 230]+0)/383;c3 = ([120 150 230]+128)/383;patch([0 1 1 0],[0 0 1 1],c1);patch([0 1 1 1-e 1-e 0+e],[0 0 1 1-e 0+e 0+e],c2);patch([0 0 1 1-e 0+e 0+e],[0 1 1 1-e 1-e 0+e],c3);plot([0 1 1 0 0],[0 0 1 1 0]);disp('W');
  "b{1}" : Constant  Value=[-1.5245225286757662086500886289286427199840545654296875;1.6058316686755433888578181722550652921199798583984375;1.517403103952690290867622024961747229099273681640625;-1.386904812575269207997052944847382605075836181640625;-1.3545623995403683892391200060956180095672607421875;1.470857444827213367233298413339070975780487060546875;-1.2857387543680351971175923608825542032718658447265625;-1.359082929289666452632445725612342357635498046875;-1.3064762119514614635562566036242060363292694091796875;-1.22721098835727193687716862768866121768951416015625;1.2308531077143507470594840924604795873165130615234375;1.336790839668508201754093533963896334171295166015625;1.11248789445838536238397864508442580699920654296875;1.161779163995248609353438951075077056884765625;-1.11085814127999693567971917218528687953948974609375;-1.16588845394895290752401706413365900516510009765625;0.978431286318926396461392869241535663604736328125;-1.0267597507064201156623539645806886255741119384765625;-1.0466534182444442446779930833145044744014739990234375;1.05098808141578725638964897370897233486175537109375;0.93621859385301731126816093819797970354557037353515625;-1.000511208787383310436780448071658611297607421875;-0.90766483038739564914720858723740093410015106201171875;-0.84546048837210940885000809430493973195552825927734375;0.84876630264789287849680476938374340534210205078125;-0.80185690636105755313423060215427540242671966552734375;-0.5148210028828319462235185710596852004528045654296875;-0.65524102483332169466478944741538725793361663818359375;0.715828663178128099531249972642399370670318603515625;0.547477588095126588285666002775542438030242919921875;0.6337090972519561216103056722204200923442840576171875;0.61282296794795898531305056167184375226497650146484375;-0.62963945517072217317178228768170811235904693603515625;-0.5600633886452470733274822123348712921142578125;-0.5142547132588661806806840104400180280208587646484375;0.36622414618450871426347248416277579963207244873046875;0.435171860018647882473175059203640557825565338134765625;-0.3973775967826436161800529589527286589145660400390625;-0.412985049052973895999940623369184322655200958251953125;-0.456498738819200500227424299737322144210338592529296875;-0.368563532068655719253769120768993161618709564208984375;-0.1451264394857011696959858682021149434149265289306640625;0.2374280696468461793191551123527460731565952301025390625;0.169516230719349125788397714131860993802547454833984375;-0.01207776799942027710910164017832357785664498805999755859375;0.07982326989852468746011737721346435137093067169189453125;0.18978690166193568078512043939554132521152496337890625;0.1312090183858221903445695488699129782617092132568359375;-0.13599776027038201764440827901125885546207427978515625;0.0259802672083776220457451699985540471971035003662109375;0.09588393978311908483203040987064014188945293426513671875;-0.000439077264281844520908693052518856347887776792049407958984375;0.10623277174090879626522365697383065707981586456298828125;-0.1382214176826130069830611546422005631029605865478515625;0.128992117787592286415332409887923859059810638427734375;-0.0820858742952841613504944007218000479042530059814453125;-0.1798165459899483398231723185745067894458770751953125;-0.386315691932279381415327179638552479445934295654296875;0.18505331061093144295881529615144245326519012451171875;-0.276070952220042686864331926699378527700901031494140625;0.1470903025261399432732645209398469887673854827880859375;0.355437619732055509746970756168593652546405792236328125;-0.33831043495201262860661017839447595179080963134765625;-0.507272391830840607696018196293152868747711181640625;0.459441289358410720478076427752966992557048797607421875;0.424515668838529147688376497171702794730663299560546875;0.63498576332306655434223330303211696445941925048828125;0.487893153924136402377342847103136591613292694091796875;0.69410429992965394507820064973202534019947052001953125;0.751872227891053679371680118492804467678070068359375;-0.82872934292105782105863909237086772918701171875 ...(+1580 chars)]
      mask Display: e = 0.06;c1 = [120 150 230]/255;c2 = ([120 150 230]+0)/383;c3 = ([120 150 230]+128)/383;patch([0 1 1 0],[0 0 1 1],c1);patch([0 1 1 1-e 1-e 0+e],[0 0 1 1-e 0+e 0+e],c2);patch([0 0 1 1-e 0+e 0+e],[0 1 1 1-e 1-e 0+e],c3);plot([0 1 1 0 0],[0 0 1 1 0]);disp('b');
  netsum : Sum  Inputs=2  SaturateOnIntegerOverflow=on  InputSameDT=on  OutDataTypeStr=Inherit: Same as first input
      mask Display: e = 0.06;c1 = [120 150 230]/255;c2 = ([120 150 230]+0)/383;c3 = ([120 150 230]+128)/383;patch([0 1 1 0],[0 0 1 1],c1);patch([0 1 1 1-e 1-e 0+e],[0 0 1 1-e 0+e 0+e],c2);patch([0 0 1 1-e 0+e 0+e],[0 1 1 1-e 1-e 0+e],c3);plot([0 1 1 0 0],[0 0 1 1 0]);disp('+');
  tansig : neural/Transfer Functions/tansig
  "a{1}" : Outport  InitialOutput=[0;0;0;0;0;0;0;0;0;0;0;0;0;0;0;0;0;0;0;0;0;0;0;0;0;0;0;0;0;0;0;0;0;0;0;0;0;0;0;0;0;0;0;0;0;0;0;0;0;0;0;0;0;0;0;0;0;0;0;0;0;0;0;0;0;0;0;0;0;0;0;0;0;0;0;0;0;0;0;0;0;0;0;0;0;0;0;0;0;0;0;0;0;0;0;0;0;0;0;0]
      mask Display: e = 0.06;c1 = [120 230 180]/255;c2 = ([120 230 180]+0)/(256+128);c3 = ([120 230 180]+128)/(256+128);patch([0 1 1 0],[0 0 1 1],c1);patch([0 1 1 1-e 1-e 0+e],[0 0 1 1-e 0+e 0+e],c2);patch([0 0 1 1-e 0+e 0+e],[0 1 1 1-e 1-e 0+e],c3);plot([0 1 1 0 0],[0 0 1 1 0]);
  wires:
  "p{1}"/1 -> Delays 1/1("p{1}")
  Delays 1/1("pd{1,1}") -> "IW{1,1}"/1("pd{1,1}")
  "IW{1,1}"/1("iz{1,1}") -> netsum/1
  "b{1}"/1 -> netsum/2
  netsum/1 -> tansig/1
  tansig/1 -> "a{1}"/1
